simulink model "Quadrotor_Model_Pitch"  (R2016a)
settings: Solver=VariableStepAuto  StartTime=0.0  StopTime=20  RelTol=1e-3
settings Model: Creator=SRQ  LastModifiedBy=SRQ

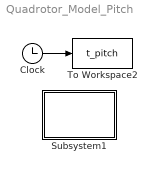
== system Quadrotor_Model_Pitch ==
  Clock : Clock
  Subsystem1 : Subsystem
      mask Display: disp('俯仰通道');
  To Workspace2 : ToWorkspace  VariableName=t_pitch  SampleTime=-1
  wires:
  Clock/1 -> To Workspace2/1

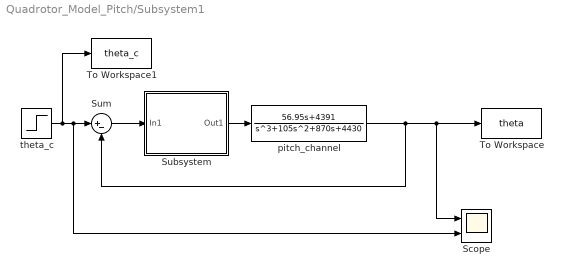
== system Quadrotor_Model_Pitch/Subsystem1 ==
  Scope : Scope  NumInputPorts=2
  Subsystem : Subsystem  mask{kp=1, ki=5, kd=0.01}
      mask Display: disp('PID');
  Sum : Sum  Inputs=|+-
  To Workspace : ToWorkspace  VariableName=theta  SampleTime=-1
  To Workspace1 : ToWorkspace  VariableName=theta_c  SampleTime=-1
  pitch_channel : TransferFcn  Numerator=[56.95 4391]  Denominator=[1 105 870 4430]
  theta_c : Step  Time=0  SampleTime=0
  wires:
  Sum/1 -> Subsystem/1(In1)
  Subsystem/1(Out1) -> pitch_channel/1
  pitch_channel/1 -> Sum/2, Scope/1, To Workspace/1
  theta_c/1 -> To Workspace1/1, Scope/2, Sum/1

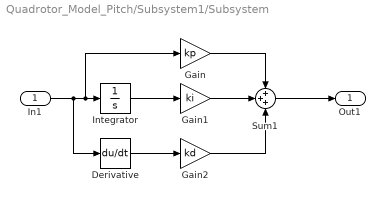
== system Quadrotor_Model_Pitch/Subsystem1/Subsystem ==
  In1 : Inport
  Derivative : Derivative
  Gain : Gain  Gain=kp
  Gain1 : Gain  Gain=ki
  Gain2 : Gain  Gain=kd
  Integrator : Integrator
  Sum1 : Sum  Inputs=+++
  Out1 : Outport
  wires:
  Integrator/1 -> Gain1/1
  Derivative/1 -> Gain2/1
  Gain2/1 -> Sum1/3
  Gain/1 -> Sum1/1
  In1/1 -> Derivative/1, Gain/1, Integrator/1
  Sum1/1 -> Out1/1
  Gain1/1 -> Sum1/2
